simulink model "sync_gen2_test"  (Simulink 7.0)
settings: Solver=ode45  StartTime=0.0  StopTime=1000  RelTol=1e-3
undefined symbols (not defined in the file): isi_correlator_lib, sync_gen2
libraries: xbsIndex_r4 x22, xps_library x6, casper_library x4
settings Model: Creator=wjm  LastModifiedBy=wjm

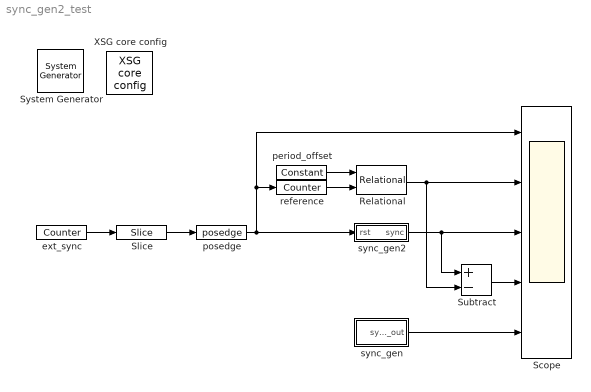
== system sync_gen2_test ==
  " System Generator" : xbsIndex_r4/ System Generator  Tag=genX  SystemSampleTime=-1  xilinxfamily=virtex5  part=xc5vsx95t  speed=-1  package=ff1136  synthesis_tool=XST  clock_wrapper=Clock Enables  directory=./isi_correlator_cropped/sysgen  testbench=off  simulink_period=1  sysclk_period=5  dcm_input_clock_period=100  incr_netlist=off  trim_vbits=Everywhere in SubSystem  dbl_ovrd=According to Block Masks  core_generation=According to Block Masks  run_coregen=off  deprecated_control=off  eval_field=0  block_type=sysgen
      settings: block_version=10.1.1
  Relational : xbsIndex_r4/Relational  mode=a=b  en=off  latency=0  dbl_ovrd=off  block_type=relational
      settings: block_version=10.1.3
  Scope : Scope  NumInputPorts=5
      settings: YMin=-5~-5~-5~-5~-5  YMax=5~5~5~5~5
  Slice : xbsIndex_r4/Slice  nbits=1  boolean_output=on  mode=Upper Bit Location + Width  bit1=0  base1=MSB of Input  bit0=0  base0=LSB of Input  dbl_ovrd=off  block_type=slice
      settings: infoedit="Extracts a given range of bits from each input sample and presents it at the output.  The output type is ordinarily unsigned with binary point at zero, but can be Boolean when the slice is one bit wide.<P><P>Hardware notes: In hardware this block costs nothing."  block_version=10.1.3
  Subtract : Sum  Inputs=+-  OutDataType=sfix(16)  OutScaling=2^-10
  XSG core config : xps_library/XSG core config  Tag=xps:xsg  SystemSampleTime=-1  hw_sys=ROACH:sx95t  ibob_linux=off  clk_src=adc0_clk  iBOB_clk_src=sys_clk  BEE2_ctrl_clk_src=sys_clk  BEE2_usr_clk_src=sys_clk  ROACH_clk_src=adc0_clk  CORR_clk_src=sys_clk  gpio_clk_io_group=iBOB:sma  gpio_clk_bit_index=0  clk_rate=200  sample_period=1  synthesis_tool=XST  mpc_type=powerpc440_ext
  ext_sync : xbsIndex_r4/Counter  cnt_type=Free Running  cnt_to=Inf  operation=Up  start_count=0  cnt_by_val=1  arith_type=Unsigned  n_bits=8  bin_pt=0  load_pin=off  rst=off  en=off  explicit_period=on  period=1  dbl_ovrd=off  use_behavioral_HDL=off  use_rpm=off  implementation=Fabric  block_type=counter
  period_offset : xbsIndex_r4/Constant  arith_type=Unsigned  const=0  n_bits=3  bin_pt=0  explicit_period=on  period=1  equ=P=C  opselect=C  inp2=PCIN>>17  opr=+  inp1=P  carry=CIN  dbl_ovrd=off  block_type=constant
      settings: block_version=10.1.1
  posedge : casper_library/Misc/posedge  Tag=Rising Edge Detector  SystemSampleTime=-1
  reference : xbsIndex_r4/Counter  cnt_type=Free Running  cnt_to=Inf  operation=Up  start_count=0  cnt_by_val=1  arith_type=Unsigned  n_bits=3  bin_pt=0  load_pin=off  rst=on  en=off  explicit_period=on  period=1  dbl_ovrd=off  use_behavioral_HDL=off  use_rpm=off  implementation=Fabric  block_type=counter
  sync_gen : Subsystem  AncestorBlock=casper_library/Misc/sync_gen  mask(sync_gen){sim_acc_len=1, fft_size=6, fft_simult_inputs=1, pfb_fir_taps=1, reorder_vec=1, scale=1}
      mask prompts: sim_acc_len "Simulation Accumulation Length"; fft_size "FFT Size"; fft_simult_inputs "Simultaneous Inputs (FFT)"; pfb_fir_taps "Taps in pfb_fir (use 1 if no pfb_fir)"; reorder_vec "Reorder Orders (e.g. [2 2 2])"
      mask help:
      | This block computes the sync period based on system parameters as
      | described in Casper memo.  Detailed descritions of the block's
      | variables can be found in the 'Block Documentation' section of
      | the CASPER wiki.
      mask init:
      | sync_gen_init(gcb, ...
      |     'sim_acc_len', sim_acc_len, ...
      |     'fft_size', fft_size, ...
      |     'fft_simult_inputs', fft_simult_inputs,...
      |     'pfb_fir_taps', pfb_fir_taps, ...
      |     'reorder_vec', reorder_vec, ...
      |     'scale', scale);
      settings: AttributesFormatString=sim_sync_period=6
      mask Help:
      | SyncPeriod=LCM(reorder_vec)*(acc_num)*(pfb_fir_len)*(fft_size/fft_simult_inputs)
      | 
      | See CASPER sync pulse memo for more details.
  sync_gen2 : Subsystem  AncestorBlock=isi_correlator_lib/sync_gen2  mask(sync_gen2){using_pfb_fir=off, pfb_fir_taps=1, using_fft=on, fft_size=7, fft_inputs=4, fft_orders=1, using_ct=off, ct_type=Double-buffered, using_vacc=off, vacc_length=0, using_scale_factor=off, scale_factor=1}
      mask prompts: using_pfb_fir "This design uses a PFB FIR."; pfb_fir_taps "Number of taps in PFB FIR:"; using_fft "This design uses an FFT."; fft_size "Size of FFT: (2^?)"; fft_inputs "Number of FFT inputs: (2^?)"; fft_orders "Order of FFT reorders: (vector)"; using_ct "This design uses a corner turner."; ct_type "Type of reorder operation:"; using_vacc "This design uses a vector accumulator."; vacc_length "Length of accumulations: (2^?)"; using_scale_factor "Scale the minimum period by an arbitrary amount."; scale_factor "Scale factor:"
      mask help: This block generates a sync pulse of an appropriate period based on the specified mask parameters.
      mask init:
      | sync_gen2_init(gcb, ...
      |     'using_pfb_fir', using_pfb_fir, ...
      |     'pfb_fir_taps', pfb_fir_taps, ...
      |     'using_fft', using_fft, ...
      |     'fft_size', fft_size, ...
      |     'fft_inputs', fft_inputs, ...
      |     'fft_orders', fft_orders, ...
      |     'using_ct', using_ct, ...
      |     'ct_type', ct_type, ...
      |     'using_vacc', using_vacc, ...
      |     'vacc_length', vacc_length, ...
      |     'using_scale_factor', using_scale_factor, ...
      |     'scale_factor', scale_factor);
      settings: AttributesFormatString=sync_period=8
      mask StyleString: checkbox,edit,checkbox,edit,edit,edit,checkbox,popup(Double-buffered|In-place),checkbox,edit,checkbox,edit
      mask CallbackString:
      | thisVariable = 'using_pfb_fir';
      | affectedVars = {'pfb_fir_taps'};
      | 
      | thisBlock = gcb();
      | thisVarState = get_param(thisBlock, thisVariable);
      | maskNames = get_param(thisBlock, 'MaskNames');
      | maskEnables = get_param(thisBlock, 'MaskEnables');
      | 
      | for varName = affectedVars
      |     varIndex = find(ismember(maskNames, varName));
      |     maskEnables{varIndex} = thisVarState;
      | end
      | 
      | set_param(thisBlock, 'MaskEnables', maskEnables);||thisVariable = 'using_fft';
      | affectedVars = {'fft_size', 'fft_inputs', 'fft_orders'};
      | 
      | thisBlock = gcb();
      | thisVarState = get_param(thisBlock, thisVariable);
      | maskNames = get_param(thisBlock, 'MaskNames');
      | maskEnables = get_param(thisBlock, 'MaskEnables');
      | 
      | for varName = affectedVars
      |     varIndex = find(ismember(maskNames, varName));
      |     maskEnables{varIndex} = thisVarState;
      | end
      | 
      | set_param(thisBlock, 'MaskEnables', maskEnables);||||thisVariable = 'using_ct';
      | affectedVars = {'ct_type'};
      | 
      | thisBlock = gcb();
      | thisVarState = get_param(thisBlock, thisVariable);
      | maskNames = get_param(thisBlock, 'MaskNames');
      | maskEnables = get_param(thisBlock, 'MaskEnables');
      | 
      | for varName = affectedVars
      |     varIndex = find(ismember(maskNames, varName));
      |     maskEnables{varIndex} = thisVarState;
      | end
      | 
      | set_param(thisBlock, 'MaskEnables', maskEnables);||thisVariable = 'using_vacc';
      | affectedVars = {'vacc_length'};
      | 
      | thisBlock = gcb();
      | thisVarState = get_param(thisBlock, thisVariable);
      | maskNames = get_param(thisBlock, 'MaskNames');
      | maskEnables = get_param(thisBlock, 'MaskEnables');
      | 
      | for varName = affectedVars
      |     varIndex = find(ismember(maskNames, varName));
      |     maskEnables{varIndex} = thisVarState;
      | end
      | 
      | set_param(thisBlock, 'MaskEnables', maskEnables);||thisVariable = 'using_scale_factor';
      | affectedVars = {'scale_factor'};
      | 
      | thisBlock = gcb();
      | thisVarState = get_param(thisBlock, thisVariable);
      | maskNames = get_param(thisBlock, 'MaskNames');
      | maskEnables = get_param(thisBlock, 'MaskEnables');
      | 
      | for varName = affectedVars
      |     varIndex = find(ismember(maskNames, varName));
      |     maskEnables{varIndex} = thisVarState;
      | end
      | 
      | set_param(thisBlock, 'MaskEnables', maskEnables);|
  wires:
  ext_sync/1 -> Slice/1
  Slice/1 -> posedge/1
  posedge/1 -> sync_gen2/1(rst), reference/1, Scope/1
  sync_gen2/1(sync) -> Subtract/1, Scope/3
  period_offset/1 -> Relational/1
  reference/1 -> Relational/2
  Relational/1 -> Subtract/2, Scope/2
  Subtract/1 -> Scope/4
  sync_gen/1(sync_out) -> Scope/5

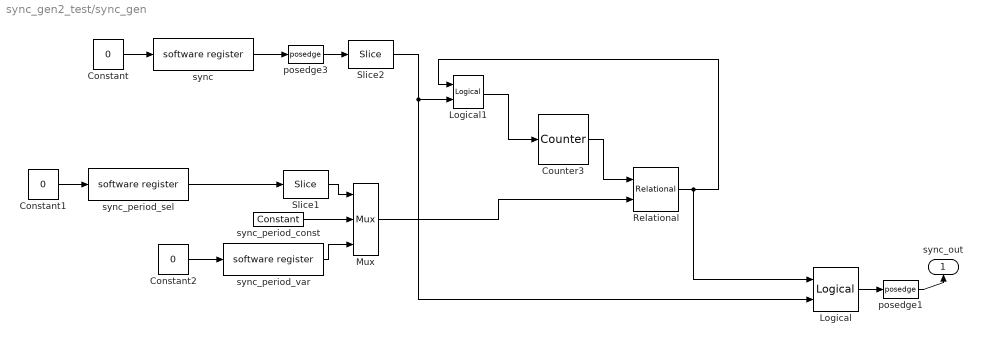
== system sync_gen2_test/sync_gen ==
  Constant : Constant  Value=0  OutDataType=sfix(16)  OutScaling=2^0
  Constant1 : Constant  Value=0  OutDataType=sfix(16)  OutScaling=2^0
  Constant2 : Constant  Value=0  OutDataType=sfix(16)  OutScaling=2^0
  Counter3 : xbsIndex_r4/Counter  cnt_type=Free Running  cnt_to=Inf  operation=Up  start_count=0  cnt_by_val=1  arith_type=Unsigned  n_bits=32  bin_pt=0  load_pin=off  rst=on  en=off  explicit_period=on  period=1  dbl_ovrd=off  use_behavioral_HDL=off  use_rpm=on  implementation=Fabric  block_type=counter
      settings: xl_area=[0, 0, 0, 0, 0, 0, 0]
  Logical : xbsIndex_r4/Logical  logical_function=OR  inputs=2  en=off  latency=0  precision=Full  arith_type=Unsigned  n_bits=8  bin_pt=2  align_bp=on  dbl_ovrd=off  block_type=logical
      settings: xl_area=[0, 0, 0, 0, 0, 0, 0]
  Logical1 : xbsIndex_r4/Logical  logical_function=OR  inputs=2  en=off  latency=0  precision=Full  arith_type=Unsigned  n_bits=8  bin_pt=2  align_bp=on  dbl_ovrd=off  block_type=logical
      settings: xl_area=[0, 0, 0, 0, 0, 0, 0]
  Mux : xbsIndex_r4/Mux  inputs=2  en=off  latency=0  precision=Full  arith_type=Unsigned  n_bits=16  bin_pt=14  quantization=Truncate  overflow=Wrap  dbl_ovrd=off  block_type=mux
  Relational : xbsIndex_r4/Relational  mode=a=b  en=off  latency=1  dbl_ovrd=off  block_type=relational
      settings: xl_area=[0, 0, 0, 0, 0, 0, 0]  block_version=10.1.3
  Slice1 : xbsIndex_r4/Slice  nbits=1  boolean_output=on  mode=Lower Bit Location + Width  bit1=0  base1=MSB of Input  bit0=0  base0=LSB of Input  dbl_ovrd=off  block_type=slice
      settings: infoedit="Extracts a given range of bits from each input sample and presents it at the output.  The output type is ordinarily unsigned with binary point at zero, but can be Boolean when the slice is one bit wide.<P><P>Hardware notes: In hardware this block costs nothing."  block_version=10.1.3
  Slice2 : xbsIndex_r4/Slice  nbits=1  boolean_output=on  mode=Lower Bit Location + Width  bit1=0  base1=MSB of Input  bit0=0  base0=LSB of Input  dbl_ovrd=off  block_type=slice
      settings: infoedit="Extracts a given range of bits from each input sample and presents it at the output.  The output type is ordinarily unsigned with binary point at zero, but can be Boolean when the slice is one bit wide.<P><P>Hardware notes: In hardware this block costs nothing."  block_version=10.1.3
  posedge1 : casper_library/Misc/posedge  Tag=Rising Edge Detector  SystemSampleTime=-1
  posedge3 : casper_library/Misc/posedge  Tag=Rising Edge Detector  SystemSampleTime=-1
  sync : xps_library/software register  Tag=xps:sw_reg  SystemSampleTime=-1  io_dir=From Processor  arith_type=Unsigned  bitwidth=32  bin_pt=0  sample_period=1  gw_name=sync_gen2_test_sync_gen_sync_user_data_out
      link override sync_gen2_test_sync_gen_sync_user_data_out: arith_type=Unsigned  n_bits=32  bin_pt=0  period=1
  sync_period_const : xbsIndex_r4/Constant  arith_type=Signed (2's comp)  const=6  n_bits=32  bin_pt=0  explicit_period=off  period=1  equ=P=C  opselect=C  inp2=PCIN>>17  opr=+  inp1=P  carry=CIN  dbl_ovrd=off  block_type=constant
      settings: block_version=10.1.1
  sync_period_sel : xps_library/software register  Tag=xps:sw_reg  SystemSampleTime=-1  io_dir=From Processor  arith_type=Unsigned  bitwidth=32  bin_pt=0  sample_period=1  gw_name=sync_gen2_test_sync_gen_sync_period_sel_user_data_out
      link override sync_gen2_test_sync_gen_sync_period_sel_user_data_out: arith_type=Unsigned  n_bits=32  bin_pt=0  period=1
  sync_period_var : xps_library/software register  Tag=xps:sw_reg  SystemSampleTime=-1  io_dir=From Processor  arith_type=Unsigned  bitwidth=32  bin_pt=0  sample_period=1  gw_name=sync_gen2_test_sync_gen_sync_period_var_user_data_out
      link override sync_gen2_test_sync_gen_sync_period_var_user_data_out: arith_type=Unsigned  n_bits=32  bin_pt=0  period=1
  sync_out : Outport  Orientation=up  OutDataType=sfix(16)  OutScaling=2^0
  wires:
  Constant/1 -> sync/1
  sync/1 -> posedge3/1
  posedge3/1 -> Slice2/1
  Logical1/1 -> Counter3/1
  Relational/1 -> Logical/1, Logical1/1
  Logical/1 -> posedge1/1
  posedge1/1 -> sync_out/1
  Constant1/1 -> sync_period_sel/1
  sync_period_sel/1 -> Slice1/1
  Slice1/1 -> Mux/1
  sync_period_const/1 -> Mux/2
  sync_period_var/1 -> Mux/3
  Constant2/1 -> sync_period_var/1
  Counter3/1 -> Relational/1
  Mux/1 -> Relational/2
  Slice2/1 -> Logical1/2, Logical/2

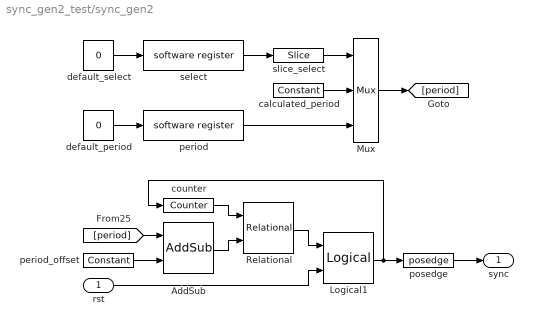
== system sync_gen2_test/sync_gen2 ==
  rst : Inport  OutDataType=sfix(16)  OutScaling=2^0
  AddSub : xbsIndex_r4/AddSub  mode=Subtraction  use_carryin=off  use_carryout=off  en=off  latency=2  precision=Full  arith_type=Unsigned  n_bits=16  bin_pt=14  quantization=Truncate  overflow=Wrap  dbl_ovrd=off  use_behavioral_HDL=off  pipelined=off  use_rpm=on  hw_selection=Fabric  block_type=addsub
      settings: block_version=10.1.3
  Logical1 : xbsIndex_r4/Logical  logical_function=OR  inputs=2  en=off  latency=0  precision=Full  arith_type=Unsigned  n_bits=16  bin_pt=0  align_bp=on  dbl_ovrd=off  block_type=logical
  Mux : xbsIndex_r4/Mux  inputs=2  en=off  latency=0  precision=Full  arith_type=Unsigned  n_bits=16  bin_pt=14  quantization=Truncate  overflow=Wrap  dbl_ovrd=off  block_type=mux
  Relational : xbsIndex_r4/Relational  mode=a>=b  en=off  latency=1  dbl_ovrd=off  block_type=relational
      settings: block_version=10.1.3
  calculated_period : xbsIndex_r4/Constant  arith_type=Unsigned  const=8  n_bits=32  bin_pt=0  explicit_period=on  period=1  equ=P=C  opselect=C  inp2=PCIN>>17  opr=+  inp1=P  carry=CIN  dbl_ovrd=off  block_type=constant
      settings: block_version=10.1.1
  counter : xbsIndex_r4/Counter  cnt_type=Free Running  cnt_to=Inf  operation=Up  start_count=0  cnt_by_val=1  arith_type=Unsigned  n_bits=32  bin_pt=0  load_pin=off  rst=on  en=off  explicit_period=on  period=1  dbl_ovrd=off  use_behavioral_HDL=off  use_rpm=off  implementation=Fabric  block_type=counter
  default_period : Constant  Value=0  OutDataType=sfix(16)  OutScaling=2^0  SampleTime=1
  default_select : Constant  Value=0  OutDataType=sfix(16)  OutScaling=2^0  SampleTime=1
  period : xps_library/software register  Tag=xps:sw_reg  SystemSampleTime=-1  io_dir=From Processor  arith_type=Unsigned  bitwidth=32  bin_pt=0  sample_period=1  gw_name=sync_gen2_test_sync_gen2_period_user_data_out
      link override isi_spectrometer_cropped_sync_gen2_period_user_data_out: arith_type=Unsigned  n_bits=32  bin_pt=0  period=1
      link override sync_gen2_test_sync_gen2_period_user_data_out: arith_type=Unsigned  n_bits=32  bin_pt=0  period=1
      link override untitled1_sync_gen2_period_user_data_out: arith_type=Unsigned  n_bits=32  bin_pt=0  period=1
  period_offset : xbsIndex_r4/Constant  arith_type=Unsigned  const=3  n_bits=32  bin_pt=0  explicit_period=on  period=1  equ=P=C  opselect=C  inp2=PCIN>>17  opr=+  inp1=P  carry=CIN  dbl_ovrd=off  block_type=constant
      settings: block_version=10.1.1
  posedge : casper_library/Misc/posedge  Tag=Rising Edge Detector  SystemSampleTime=-1
  select : xps_library/software register  Tag=xps:sw_reg  SystemSampleTime=-1  io_dir=From Processor  arith_type=Unsigned  bitwidth=32  bin_pt=0  sample_period=1  gw_name=sync_gen2_test_sync_gen2_select_user_data_out
      link override isi_spectrometer_cropped_sync_gen2_select_user_data_out: arith_type=Unsigned  n_bits=32  bin_pt=0  period=1
      link override sync_gen2_test_sync_gen2_select_user_data_out: arith_type=Unsigned  n_bits=32  bin_pt=0  period=1
      link override untitled1_sync_gen2_select_user_data_out: arith_type=Unsigned  n_bits=32  bin_pt=0  period=1
  slice_select : xbsIndex_r4/Slice  nbits=1  boolean_output=on  mode=Lower Bit Location + Width  bit1=0  base1=MSB of Input  bit0=0  base0=LSB of Input  dbl_ovrd=off  block_type=slice
      settings: infoedit="Extracts a given range of bits from each input sample and presents it at the output.  The output type is ordinarily unsigned with binary point at zero, but can be Boolean when the slice is one bit wide.<P><P>Hardware notes: In hardware this block costs nothing."  block_version=10.1.3
  sync : Outport  OutDataType=sfix(16)  OutScaling=2^0
  wires:
  Mux/1 -> [period]
  period/1 -> Mux/3
  calculated_period/1 -> Mux/2
  slice_select/1 -> Mux/1
  default_period/1 -> period/1
  select/1 -> slice_select/1
  default_select/1 -> select/1
  [period] -> AddSub/1
  period_offset/1 -> AddSub/2
  AddSub/1 -> Relational/2
  counter/1 -> Relational/1
  Logical1/1 -> posedge/1, counter/1
  posedge/1 -> sync/1
  Relational/1 -> Logical1/1
  rst/1 -> Logical1/2
